simulink model "complete_param"  (Simulink 7.4)
settings: Solver=ode45  StartTime=0.0  StopTime=50  RelTol=1e-3
values from neighbouring files (symbols this model uses):
  phi0 = 0.15    [Quadrocopter_control_Driver.m]    (also in calc_stability.m = 0)
  r_phi0 = 0    [Quadrocopter_control_Driver.m]    (also in calc_stability.m)
  r_psi0 = 0    [Quadrocopter_control_Driver.m]    (also in calc_stability.m)
  r_theta0 = 0    [Quadrocopter_control_Driver.m]    (also in calc_stability.m)
  theta0 = 0.15    [Quadrocopter_control_Driver.m]    (also in calc_stability.m = 0)
undefined symbols (not defined in the file or in its folder): boom, f1, f2, f3, f4, f5, I_x, I_y, I_z
libraries: Copter_Library x5
settings Model: Creator=alstit04  LastModifiedBy=Alex

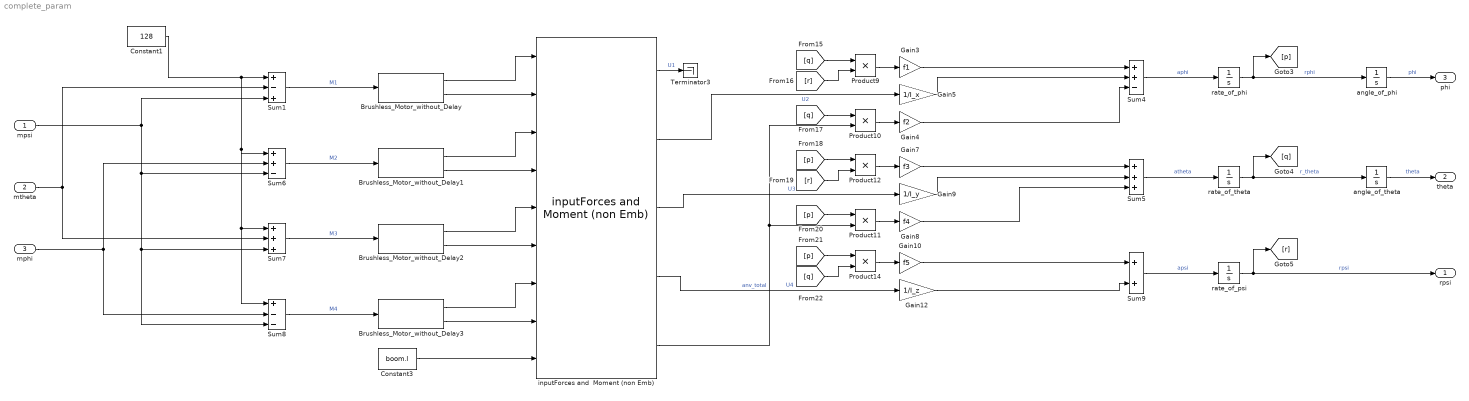
== system complete_param ==
  mpsi : Inport  OutDataType=fixdt(1, 16)  OutScaling=2^0
  mtheta : Inport  Port=2  OutDataType=fixdt(1, 16)  OutScaling=2^0
  mphi : Inport  Port=3  OutDataType=fixdt(1, 16)  OutScaling=2^0
  Brushless_Motor_without_Delay{,1..3} (4 alike) : Copter_Library/Brushless_Motor_without_Delay  SystemSampleTime=-1  M_error=0.99
  Constant1 : Constant  Value=128
  Constant3 : Constant  Value=boom.l
  Gain10 : Gain  Gain=f5
  Gain12 : Gain  Gain=1/I_z
  Gain3 : Gain  Gain=f1
  Gain4 : Gain  Gain=f2
  Gain5 : Gain  Gain=1/I_x
  Gain7 : Gain  Gain=f3
  Gain8 : Gain  Gain=f4
  Gain9 : Gain  Gain=1/I_y
  Product{9..12,14} (5 alike) : Product  RndMeth=Zero
  Sum1 : Sum  Inputs=+-+  OutDataType=fixdt(1, 16)  OutScaling=2^0
  Sum4 : Sum  Inputs=++-
  Sum5 : Sum  Inputs=+++
  Sum6 : Sum  Inputs=++-  OutDataType=fixdt(1, 16)  OutScaling=2^0
  Sum7 : Sum  Inputs=+++  OutDataType=fixdt(1, 16)  OutScaling=2^0
  Sum8 : Sum  Inputs=+--  OutDataType=fixdt(1, 16)  OutScaling=2^0
  Sum9 : Sum
  Terminator3 : Terminator
  angle_of_phi : Integrator  InitialCondition=phi0
  angle_of_theta : Integrator  InitialCondition=theta0
  inputForces and  Moment (non Emb) : Copter_Library/inputForces and  Moment (non Emb)  SystemSampleTime=-1
  rate_of_phi : Integrator  InitialCondition=r_phi0
  rate_of_psi : Integrator  InitialCondition=r_psi0
  rate_of_theta : Integrator  InitialCondition=r_theta0
  rpsi : Outport
  theta : Outport  Port=2
  phi : Outport  Port=3
  wires:
  Sum8/1 -> Brushless_Motor_without_Delay3/1  "M4"
  Sum6/1 -> Brushless_Motor_without_Delay1/1  "M2"
  Sum1/1 -> Brushless_Motor_without_Delay/1  "M1"
  Constant1/1 -> Sum1/1, Sum6/1, Sum7/1, Sum8/1
  Sum7/1 -> Brushless_Motor_without_Delay2/1  "M3"
  Constant3/1 -> inputForces and  Moment (non Emb)/9
  inputForces and  Moment (non Emb)/4 -> Gain12/1  "U4"
  Product14/1 -> Gain10/1
  [q] -> Product14/2
  [p] -> Product14/1
  inputForces and  Moment (non Emb)/3 -> Gain9/1  "U3"
  Product11/1 -> Gain8/1
  [p] -> Product11/1
  Product12/1 -> Gain7/1
  [r] -> Product12/2
  [p] -> Product12/1
  inputForces and  Moment (non Emb)/2 -> Gain5/1  "U2"
  Product10/1 -> Gain4/1
  [q] -> Product10/1
  Product9/1 -> Gain3/1
  [r] -> Product9/2
  [q] -> Product9/1
  inputForces and  Moment (non Emb)/5 -> Product11/2, Product10/2  "anv_total"
  Brushless_Motor_without_Delay/1 -> inputForces and  Moment (non Emb)/1
  Brushless_Motor_without_Delay/2 -> inputForces and  Moment (non Emb)/2
  Brushless_Motor_without_Delay1/1 -> inputForces and  Moment (non Emb)/3
  Brushless_Motor_without_Delay1/2 -> inputForces and  Moment (non Emb)/4
  Brushless_Motor_without_Delay2/1 -> inputForces and  Moment (non Emb)/5
  Brushless_Motor_without_Delay2/2 -> inputForces and  Moment (non Emb)/6
  Brushless_Motor_without_Delay3/1 -> inputForces and  Moment (non Emb)/7
  Brushless_Motor_without_Delay3/2 -> inputForces and  Moment (non Emb)/8
  mpsi/1 -> Sum1/3, Sum6/3, Sum7/3, Sum8/3
  mphi/1 -> Sum6/2, Sum8/2
  mtheta/1 -> Sum1/2, Sum7/2
  Sum9/1 -> rate_of_psi/1  "apsi"
  Gain12/1 -> Sum9/2
  Gain10/1 -> Sum9/1
  Sum5/1 -> rate_of_theta/1  "atheta"
  Gain9/1 -> Sum5/2
  Gain7/1 -> Sum5/1
  Sum4/1 -> rate_of_phi/1  "aphi"
  Gain5/1 -> Sum4/2
  Gain3/1 -> Sum4/1
  angle_of_phi/1 -> phi/1  "phi"
  angle_of_theta/1 -> theta/1  "theta"
  rate_of_phi/1 -> [p], angle_of_phi/1  "rphi"
  rate_of_theta/1 -> angle_of_theta/1, [q]  "r_theta"
  rate_of_psi/1 -> [r], rpsi/1  "rpsi"
  Gain4/1 -> Sum4/3
  Gain8/1 -> Sum5/3
  inputForces and  Moment (non Emb)/1 -> Terminator3/1  "U1"
